simulink model "Tip41c_test_1"  (R2024a)
settings: Solver=VariableStepAuto  StartTime=0.0  StopTime=10.0  RelTol=1e-3
libraries: arduinolib x3
settings Model: Creator=cuong  LastModifiedBy=cuong

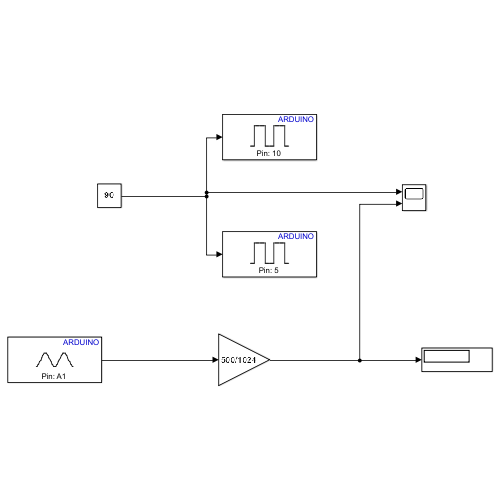
[thumbnail: Simulink's stored preview of the top-level diagram]
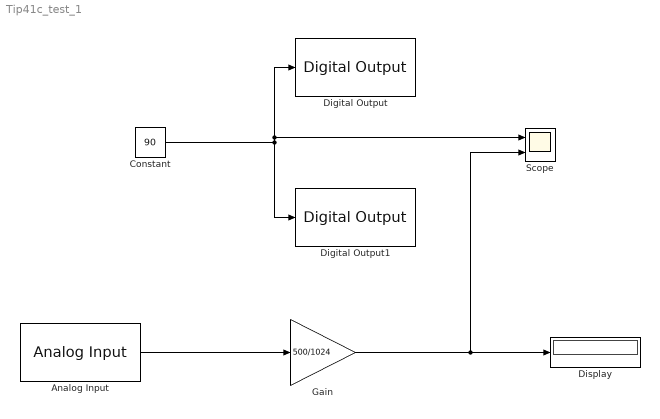
== system Tip41c_test_1 ==
  Analog Input : arduinolib/Analog Input  pinNumber=1  ReadResultsOnly=off  ConversionTriggerSource=Software  ExternalTriggerType=uint32( 0 )  OutputDataType=uint16  EnableConversionCompleteNotify=off  EnableOuputStatus=off  SampleTime=-1  blockPlatform=arduino
  Constant : Constant  Value=90
  Digital Output : arduinolib/Digital Output  pinNumber=10  Direction=output  blockPlatform=arduino
  Digital Output1 : arduinolib/Digital Output  pinNumber=5  Direction=output  blockPlatform=arduino
  Display : Display
  Gain : Gain  Gain=500/1024
  Scope : Scope  NumInputPorts=2
  wires:
  Constant/1 -> Digital Output/1, Scope/1, Digital Output1/1
  Analog Input/1 -> Gain/1
  Gain/1 -> Scope/2, Display/1
